simulink model "topic1"  (R2014a)
settings: Solver=ode45  StartTime=0.0  StopTime=0.1  RelTol=1e-3
libraries: powerlib x22, powerlib_meascontrol x5
settings Model: Creator=Administrator  LastModifiedBy=Administrator

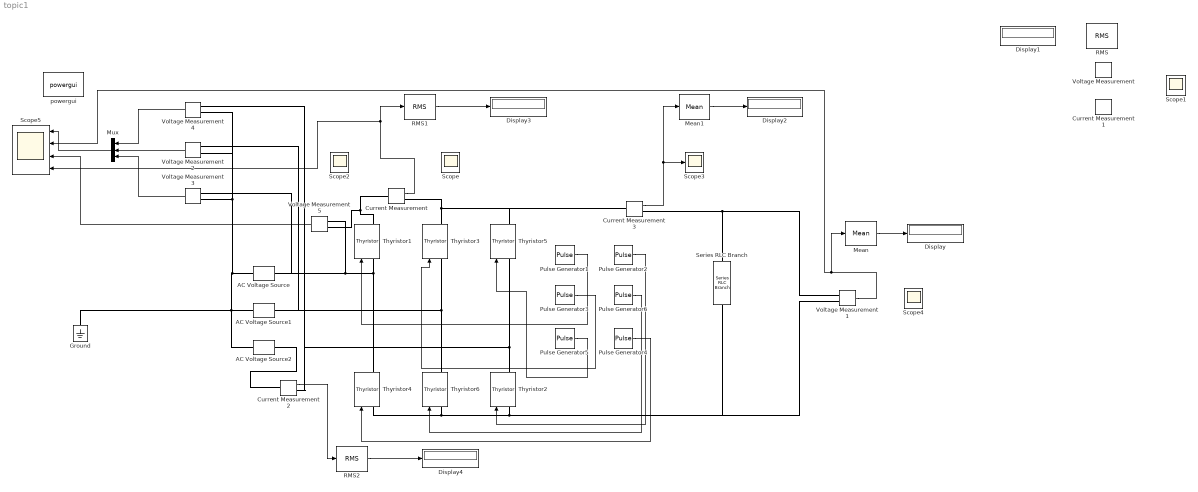
== system topic1 ==
  AC Voltage Source : powerlib/Electrical Sources/AC Voltage Source  Amplitude=311  Phase=0  Frequency=50  SampleTime=0  Measurements=None
  AC Voltage Source1 : powerlib/Electrical Sources/AC Voltage Source  Amplitude=311  Phase=240  Frequency=50  SampleTime=0  Measurements=None
  AC Voltage Source2 : powerlib/Electrical Sources/AC Voltage Source  Amplitude=311  Phase=120  Frequency=50  SampleTime=0  Measurements=None
  Current Measurement{,1..3} (4 alike) : powerlib/Measurements/Current Measurement  PhasorSimulation=off  OutputType=Complex  PSBequivalent=0
  Display{,1..4} (5 alike) : Display
  Ground : powerlib/Elements/Ground  LConnTagsString=a
  Mean : powerlib_meascontrol/Measurements/Mean  Freq=60  Vinit=0  Ts=0
  Mean1 : powerlib_meascontrol/Measurements/Mean  Freq=60  Vinit=0  Ts=0
  Mux : Mux  Inputs=3
  Pulse Generator1 : DiscretePulseGenerator  PulseType=Time based  Period=0.02  PulseWidth=33.3  PhaseDelay=0.02/12-0.02
  Pulse Generator2 : DiscretePulseGenerator  PulseType=Time based  Period=0.02  PulseWidth=33.3  PhaseDelay=0.02/4-0.02
  Pulse Generator3 : DiscretePulseGenerator  PulseType=Time based  Period=0.02  PulseWidth=33.3  PhaseDelay=0.02*5/12-0.02
  Pulse Generator4 : DiscretePulseGenerator  PulseType=Time based  Period=0.02  PulseWidth=33.3  PhaseDelay=0.02*7/12-0.02
  Pulse Generator5 : DiscretePulseGenerator  PulseType=Time based  Period=0.02  PulseWidth=33.3  PhaseDelay=0.02*3/4-0.02
  Pulse Generator6 : DiscretePulseGenerator  PulseType=Time based  Period=0.02  PulseWidth=33.3  PhaseDelay=0.02*11/12-0.02
  RMS : powerlib_meascontrol/Measurements/RMS  TrueRMS=on  Freq=50  RMSInit=120  Ts=0
  RMS1 : powerlib_meascontrol/Measurements/RMS  TrueRMS=on  Freq=50  RMSInit=120  Ts=0
  RMS2 : powerlib_meascontrol/Measurements/RMS  TrueRMS=on  Freq=50  RMSInit=120  Ts=0
  Scope{,1..4} (5 alike) : Scope
      Scope2 settings: SaveName=ScopeData2
      Scope3 settings: SaveName=ScopeData3
      Scope4 settings: SaveName=ScopeData4
  Scope5 : Scope  NumInputPorts=4
      settings: TimeRange=0.1  YMin=-400~-5~-5~-5  YMax=400~5~5~5  SaveName=ScopeData5
  Series RLC Branch : powerlib/Elements/Series RLC Branch  LConnTagsString=__new0  RConnTagsString=__new0  BranchType=RL  Resistance=10  Inductance=1e-3  SetiL0=off  InitialCurrent=0  Capacitance=1e-6  Setx0=off  InitialVoltage=0  Measurements=None
  Thyristor{1..6} (6 alike) : powerlib/Power Electronics/Thyristor  Ron=0.001  Lon=0  Vf=0.8  IC=0  Rs=500  Cs=250e-9  Measurements=on
  Voltage Measurement{,1..5} (6 alike) : powerlib/Measurements/Voltage Measurement  PhasorSimulation=off  OutputType=Complex  PSBequivalent=0
  powergui : powerlib/powergui  Priority=1  SimulationMode=Continuous  SolverType=Tustin  SampleTime=50e-6  frequency=60  SPID=off  DisableSnubberDevices=off  DisableRonSwitches=off  DisableVfSwitches=off  SwTol=0  Interpol=off  DisplayEquations=off  Ts=0  methode=off  frequencyindice=50  Pbase=100e6  ErrMax=1e-4  Iterations=50  UnitsV=kV  UnitsW=MW  FunctionMessages=off  echomessages=off  HookPort=off  EnableUseOfTLC=off  x0status=blocks  RestoreLinks=warning  ResistiveCurrentMeasurement=off  Frange=[0:2:500]  Ylog=off  Xlog=on  ShowGrid=off  save=off  variable=ZData  structure=0  ZoomFFT=off  StartTime=0.0  cycles=1  DisplayStyle=1  fundamental=60  FreqAxis=off  MaxFrequency=1000  frequencyindicesteady=1  RmsSteady=1  display=off
  wires:
  Pulse Generator1/1 -> Thyristor1/1
  Pulse Generator3/1 -> Thyristor3/1
  Pulse Generator5/1 -> Thyristor5/1
  Pulse Generator2/1 -> Thyristor2/1
  Pulse Generator6/1 -> Thyristor6/1
  Pulse Generator4/1 -> Thyristor4/1
  Current Measurement/1 -> RMS1/1, Scope5/4
  Current Measurement3/1 -> Mean1/1, Scope3/1
  Voltage Measurement1/1 -> Mean/1, Scope5/2
  Mean/1 -> Display/1
  Mean1/1 -> Display2/1
  RMS1/1 -> Display3/1
  Current Measurement2/1 -> RMS2/1
  RMS2/1 -> Display4/1
  Voltage Measurement4/1 -> Mux/1
  Voltage Measurement2/1 -> Mux/2
  Voltage Measurement3/1 -> Mux/3
  Mux/1 -> Scope5/1
  Voltage Measurement5/1 -> Scope5/3
  connections:
  AC Voltage Source/LConn1 -- Voltage Measurement4/LConn2 -- Voltage Measurement2/LConn2 -- Voltage Measurement3/LConn2 -- Ground/LConn1 -- AC Voltage Source1/LConn1 -- AC Voltage Source2/LConn1
  Thyristor3/RConn1 -- Current Measurement3/LConn1 -- Thyristor5/RConn1 -- Current Measurement/RConn1
  Thyristor2/LConn1 -- Series RLC Branch/RConn1 -- Voltage Measurement1/LConn2 -- Thyristor4/LConn1 -- Thyristor6/LConn1
  Thyristor1/LConn1 -- Voltage Measurement5/LConn1 -- Voltage Measurement3/LConn1 -- AC Voltage Source/RConn1 -- Thyristor4/RConn1
  Thyristor3/LConn1 -- Voltage Measurement2/LConn1 -- AC Voltage Source1/RConn1 -- Thyristor6/RConn1
  Thyristor5/LConn1 -- Current Measurement2/RConn1 -- Voltage Measurement4/LConn1 -- Thyristor2/RConn1
  Thyristor1/RConn1 -- Current Measurement/LConn1 -- Voltage Measurement5/LConn2
  Current Measurement3/RConn1 -- Series RLC Branch/LConn1 -- Voltage Measurement1/LConn1
  AC Voltage Source2/RConn1 -- Current Measurement2/LConn1
